simulink model "PTSD_single_channel_local_min_max_6"  (R2019b)
settings: Solver=VariableStepAuto  StartTime=0.0  StopTime=10  RelTol=1e-3
libraries: simulink x8, dspstat3 x7, dspswit3 x1
settings Model: Creator=sbuccelli  LastModifiedBy=sbuccelli

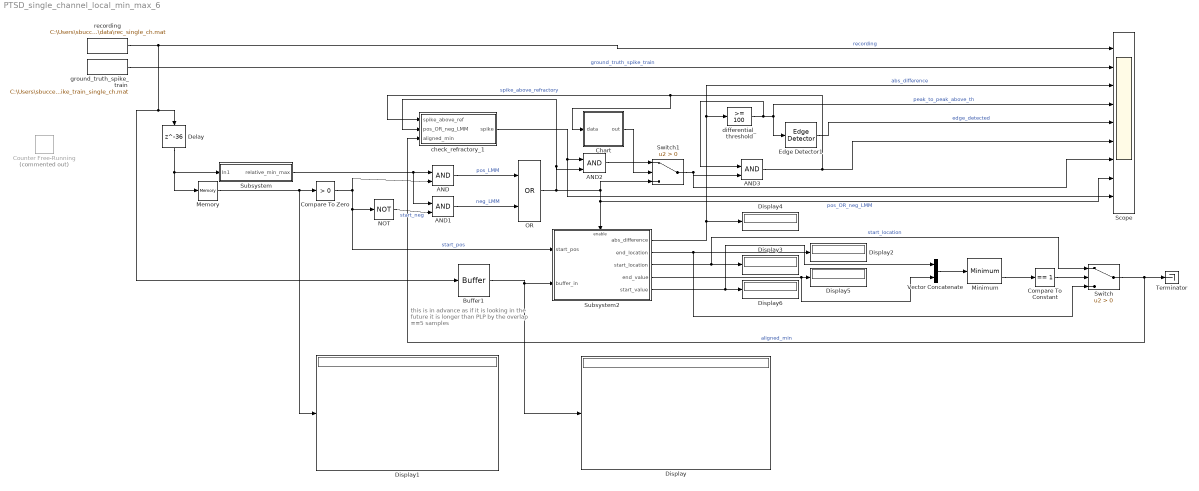
== system PTSD_single_channel_local_min_max_6 ==
  note: this is in advance as if it is looking in the future
      | it is longer than PLP by the overlap ==5 samples
  AND{,1..3} (4 alike) : Logic  IconShape=distinctive  AllPortsSameDT=off  OutDataTypeStr=boolean
  Buffer1 : Buffer  N=38  V=37  OutputFrames=off
  Chart : Stateflow chart  BlockKeywords=__PRM__SERIALIZED__DATA__:Stateflow Chart,Stateflow Diagram  TreatAsAtomicUnit=on
  Compare To Constant : simulink/Logic and Bit Operations/Compare To Constant  relop===  const=1  OutDataTypeStr=boolean
  Compare To Zero : simulink/Logic and Bit Operations/Compare To Zero  relop=>  OutDataTypeStr=boolean
  Counter Free-Running : simulink/Sources/Counter Free-Running  Commented=on  NumBits=32  tsamp=-1
  Delay : Delay  DelayLength=36
  Display{,1..6} (7 alike) : Display
  Edge Detector1 : dspswit3/Edge Detector  InputProcessing=Columns as channels (frame based)
      settings: SourceProductName=DSP System Toolbox  SourceProductBaseCode=DS
  Memory : Memory  InheritSampleTime=on
  Minimum : dspstat3/Minimum  operation=minimum  fcn=Value and Index  indexBase=One  operateOver=Each column  Dimension=1  InputProcessing=Columns as channels (frame based)  reset=None  roiEnable=off  roiType=Rectangles  roiPortion=Entire ROI  roiOutput=Individual statistics for each ROI  roiFlag=off  roundingMode=Floor  overflowMode=off
      settings: SourceProductName=DSP System Toolbox  SourceProductBaseCode=DS
  NOT : Logic  Operator=NOT  IconShape=distinctive  AllPortsSameDT=off  OutDataTypeStr=boolean
  OR : Logic  Operator=OR  IconShape=distinctive  AllPortsSameDT=off  OutDataTypeStr=boolean
  Scope : Scope  NumInputPorts=9
  Subsystem : Subsystem
  Subsystem2 : Subsystem
  Switch : Switch  Criteria=u2 > Threshold
  Switch1 : Switch  Criteria=u2 > Threshold
  Terminator : Terminator
  Vector Concatenate : Concatenate
  check_refractory_1 : Subsystem
  differential_threshold : simulink/Logic and Bit Operations/Compare To Constant  relop=>=  const=100  OutDataTypeStr=boolean
  ground_truth_spike_train : FromFile  FileName=C:\Users\sbuccelli\Documents\GitHub\closed-loop-neuroscience\data\spike_train_single_ch.mat  SampleTime=1/32e3
  recording : FromFile  FileName=C:\Users\sbuccelli\Documents\GitHub\closed-loop-neuroscience\data\rec_single_ch.mat  SampleTime=1/32e3
  wires:
  recording/1 -> Buffer1/1, Delay/1, Scope/1  "recording"
  ground_truth_spike_train/1 -> Scope/2  "ground_truth_spike_train"
  Subsystem/1(relative_min_max) -> AND/1, AND1/1
  Compare To Zero/1 -> Subsystem2/1(start_pos), NOT/1, AND/2  "start_pos"
  NOT/1 -> AND1/2  "start_neg"
  AND/1 -> OR/1  "pos_LMM"
  AND1/1 -> OR/2  "neg_LMM"
  OR/1 -> check_refractory_1/2(pos_OR_neg_LMM), AND2/2, Subsystem2/Enable, Scope/8, Switch1/3  "pos_OR_neg_LMM"
  Delay/1 -> Memory/1, Subsystem/1(In1)
  differential_threshold/1 -> AND3/1, Scope/4, Edge Detector1/1  "peak_to_peak_above_th"
  Subsystem2/1(abs_difference) -> Display4/1, Scope/3, differential_threshold/1  "abs_difference"
  Buffer1/1 -> Display/1, Subsystem2/2(buffer_in)
  Edge Detector1/1 -> Scope/5  "edge_detected"
  AND3/1 -> Scope/6, check_refractory_1/1(spike_above_ref), Chart/1(data)  "spike_above_refractory"
  Memory/1 -> Display1/1, Compare To Zero/1
  Subsystem2/2(end_location) -> Switch/3, Display2/1
  Subsystem2/4(end_value) -> Vector Concatenate/2, Display5/1
  Subsystem2/5(start_value) -> Vector Concatenate/1, Display6/1
  Subsystem2/3(start_location) -> Switch/1, Display3/1  "start_location"
  Vector Concatenate/1 -> Minimum/1
  Minimum/2 -> Compare To Constant/1
  Compare To Constant/1 -> Switch/2
  Switch/1 -> check_refractory_1/3(aligned_min), Terminator/1  "aligned_min"
  check_refractory_1/1(spike) -> Scope/9, AND2/1
  Switch1/1 -> Scope/7, AND3/2
  AND2/1 -> Switch1/1
  Chart/1(out) -> Switch1/2

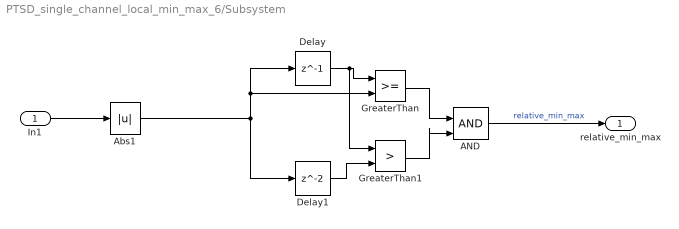
== system PTSD_single_channel_local_min_max_6/Subsystem ==
  In1 : Inport
  AND : Logic  IconShape=distinctive  AllPortsSameDT=off  OutDataTypeStr=boolean
  Abs1 : Abs
  Delay : Delay  DelayLength=1
  Delay1 : Delay
  GreaterThan : RelationalOperator  OutDataTypeStr=boolean  RndMeth=Simplest
  GreaterThan1 : RelationalOperator  Operator=>  OutDataTypeStr=boolean  RndMeth=Simplest
  relative_min_max : Outport
  wires:
  In1/1 -> Abs1/1
  Delay1/1 -> GreaterThan1/2
  GreaterThan1/1 -> AND/2
  GreaterThan/1 -> AND/1
  Delay/1 -> GreaterThan1/1, GreaterThan/1
  AND/1 -> relative_min_max/1  "relative_min_max"
  Abs1/1 -> Delay/1, GreaterThan/2, Delay1/1

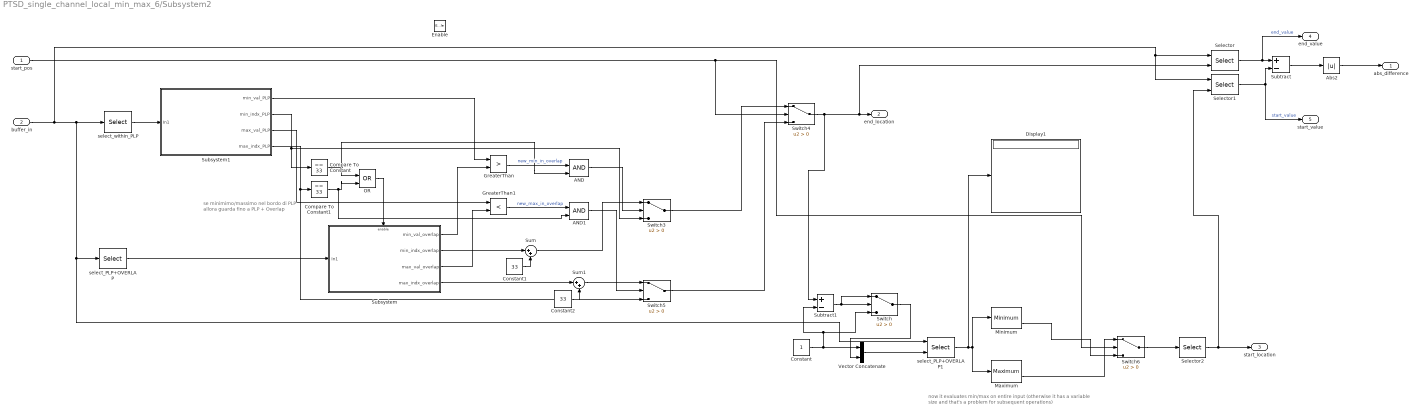
== system PTSD_single_channel_local_min_max_6/Subsystem2 ==
  note: now it evaluates min/max on entire input (otherwise it has a variable size and that's a problem for subsequent operations)
  note: se minimimo/massimo nel bordo di PLP allora guarda fino a PLP + Overlap
  start_pos : Inport
  buffer_in : Inport  Port=2
  Enable : EnablePort  PropagateVarSize=During execution
  AND : Logic  IconShape=distinctive  AllPortsSameDT=off  OutDataTypeStr=boolean
  AND1 : Logic  IconShape=distinctive  AllPortsSameDT=off  OutDataTypeStr=boolean
  Abs2 : Abs
  Compare To Constant : simulink/Logic and Bit Operations/Compare To Constant  relop===  const=33  OutDataTypeStr=boolean
  Compare To Constant1 : simulink/Logic and Bit Operations/Compare To Constant  relop===  const=33  OutDataTypeStr=boolean
  Constant : Constant
  Constant1 : Constant  Value=33
  Constant2 : Constant  Value=33
  Display1 : Display
  GreaterThan : RelationalOperator  Operator=>  OutDataTypeStr=boolean  RndMeth=Simplest
  GreaterThan1 : RelationalOperator  Operator=<  OutDataTypeStr=boolean  RndMeth=Simplest
  Maximum : dspstat3/Maximum  operation=maximum  fcn=Value and Index  indexBase=One  operateOver=Entire input  Dimension=1  InputProcessing=Columns as channels (frame based)  reset=None  roiEnable=off  roiType=Rectangles  roiPortion=Entire ROI  roiOutput=Individual statistics for each ROI  roiFlag=off  roundingMode=Floor  overflowMode=off  accumDataTypeStr=Inherit: Same as product output  accumLastDataTypeStr=Inherit: Same as product output
  Minimum : dspstat3/Minimum  operation=minimum  fcn=Value and Index  indexBase=One  operateOver=Entire input  Dimension=1  InputProcessing=Columns as channels (frame based)  reset=None  roiEnable=off  roiType=Rectangles  roiPortion=Entire ROI  roiOutput=Individual statistics for each ROI  roiFlag=off  roundingMode=Floor  overflowMode=off
      settings: SourceProductName=DSP System Toolbox  SourceProductBaseCode=DS
  OR : Logic  Operator=OR  IconShape=distinctive  AllPortsSameDT=off  OutDataTypeStr=boolean
  Selector : Selector  IndexOptions=Index vector (port)  Indices=[1 3]  OutputSizes=1
  Selector1 : Selector  IndexOptions=Index vector (port)  Indices=[1 3]  OutputSizes=1
  Selector2 : Selector  NumberOfDimensions=2  IndexOptions=Select all,Index vector (dialog)  Indices=[1 3],1  OutputSizes=1,1
  Subsystem : Subsystem
  Subsystem1 : Subsystem
  Subtract : Sum  Inputs=+-
  Subtract1 : Sum  Inputs=+-
  Sum : Sum  Inputs=|++
  Sum1 : Sum  Inputs=|++
  Switch{,3..6} (5 alike) : Switch  Criteria=u2 > Threshold
  Vector Concatenate : Concatenate
  select_PLP+OVERLAP : Selector  NumberOfDimensions=2  InputPortWidth=3  IndexOptions=Index vector (dialog),Index vector (dialog)  Indices=[34:38],1  OutputSizes=1,1
  select_PLP+OVERLAP1 : Selector  NumberOfDimensions=2  InputPortWidth=3  IndexOptions=Starting and ending indices (port),Index vector (dialog)  Indices=[25:29],1  OutputSizes=1,1
  select_within_PLP : Selector  NumberOfDimensions=2  InputPortWidth=3  IndexOptions=Index vector (dialog),Index vector (dialog)  Indices=[1:33],1  OutputSizes=1,1
  abs_difference : Outport
  end_location : Outport  Port=2
  start_location : Outport  Port=3
  end_value : Outport  Port=4
  start_value : Outport  Port=5
  wires:
  Abs2/1 -> abs_difference/1
  buffer_in/1 -> Selector1/1, Selector/1, select_within_PLP/1, select_PLP+OVERLAP1/1, select_PLP+OVERLAP/1
  Subtract/1 -> Abs2/1
  Compare To Constant/1 -> OR/1, AND/2
  Compare To Constant1/1 -> AND1/2, OR/2
  OR/1 -> Subsystem/Enable
  select_PLP+OVERLAP/1 -> Subsystem/1(In1)
  select_within_PLP/1 -> Subsystem1/1(In1)
  Subsystem1/2(min_indx_PLP) -> Switch3/3, Compare To Constant/1
  Subsystem1/4(max_indx_PLP) -> Switch5/3, Compare To Constant1/1
  Subsystem1/1(min_val_PLP) -> GreaterThan/1
  Subsystem/1(min_val_overlap) -> GreaterThan/2
  Subsystem1/3(max_val_PLP) -> GreaterThan1/1
  Subsystem/3(max_val_overlap) -> GreaterThan1/2
  GreaterThan/1 -> AND/1  "new_min_in_overlap"
  GreaterThan1/1 -> AND1/1  "new_max_in_overlap"
  AND/1 -> Switch3/2
  AND1/1 -> Switch5/2
  Switch3/1 -> Switch4/1
  Switch5/1 -> Switch4/3
  Vector Concatenate/1 -> select_PLP+OVERLAP1/2
  start_pos/1 -> Switch4/2, Switch6/2
  select_PLP+OVERLAP1/1 -> Display1/1, Maximum/1, Minimum/1
  Minimum/2 -> Switch6/3
  Maximum/2 -> Switch6/1
  Selector/1 -> end_value/1, Subtract/1  "end_value"
  Selector1/1 -> start_value/1, Subtract/2  "start_value"
  Switch4/1 -> Selector/2, end_location/1, Subtract1/1
  Switch6/1 -> Selector2/1
  Selector2/1 -> start_location/1, Selector1/2
  Subtract1/1 -> Switch/1, Switch/2
  Constant/1 -> Vector Concatenate/1, Switch/3, Subtract1/2
  Switch/1 -> Vector Concatenate/2
  Subsystem/2(min_indx_overlap) -> Sum/1
  Sum/1 -> Switch3/1
  Constant1/1 -> Sum/2
  Subsystem/4(max_indx_overlap) -> Sum1/1
  Constant2/1 -> Sum1/2
  Sum1/1 -> Switch5/1

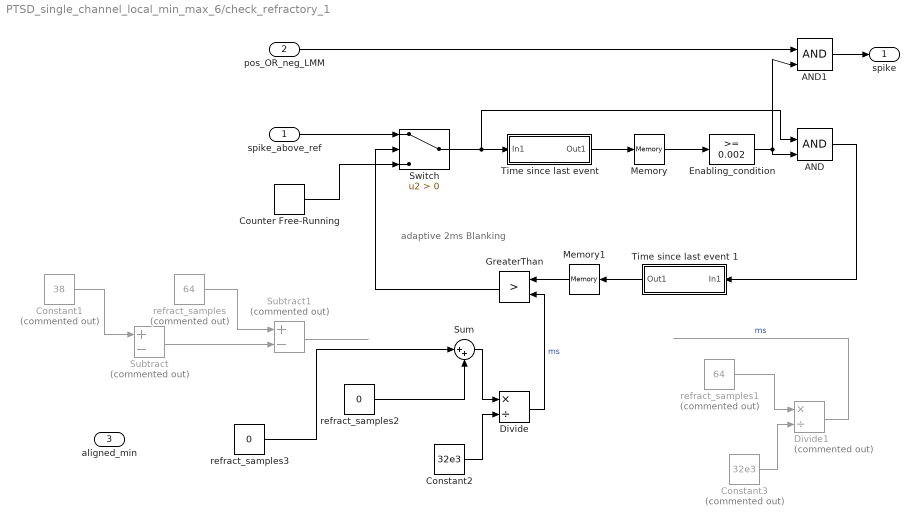
== system PTSD_single_channel_local_min_max_6/check_refractory_1 ==
  note: adaptive 2ms Blanking
  spike_above_ref : Inport
  pos_OR_neg_LMM : Inport  Port=2
  aligned_min : Inport  Port=3
  AND : Logic  IconShape=distinctive  AllPortsSameDT=off  OutDataTypeStr=boolean
  AND1 : Logic  IconShape=distinctive  AllPortsSameDT=off  OutDataTypeStr=boolean
  Constant1 : Constant  Commented=on  Value=38
  Constant2 : Constant  Value=32e3
  Constant3 : Constant  Commented=on  Value=32e3
  Counter Free-Running : simulink/Sources/Counter Free-Running  NumBits=1  tsamp=-1
  Divide : Product  Inputs=*/
  Divide1 : Product  Commented=on  Inputs=*/
  Enabling_condition : simulink/Logic and Bit Operations/Compare To Constant  relop=>=  const=0.002  OutDataTypeStr=boolean
  GreaterThan : RelationalOperator  Operator=>  OutDataTypeStr=boolean  RndMeth=Simplest
  Memory : Memory  InheritSampleTime=on
  Memory1 : Memory  InheritSampleTime=on
  Subtract : Sum  Commented=on  Inputs=+-
  Subtract1 : Sum  Commented=on  Inputs=+-
  Sum : Sum  Inputs=|++
  Switch : Switch  Criteria=u2 > Threshold
  "Time since last event " : Subsystem
  Time since last event 1 : Subsystem
  refract_samples : Constant  Commented=on  Value=64
  refract_samples1 : Constant  Commented=on  Value=64
  refract_samples2 : Constant  Value=0
  refract_samples3 : Constant  Value=0
  spike : Outport
  wires:
  Memory/1 -> Enabling_condition/1
  "Time since last event "/1(Out1) -> Memory/1
  Time since last event 1/1(Out1) -> Memory1/1
  Counter Free-Running/1 -> Switch/3
  GreaterThan/1 -> Switch/2
  spike_above_ref/1 -> Switch/1
  Switch/1 -> AND/1, "Time since last event "/1(In1)
  Constant1/1 -> Subtract/1
  Subtract/1 -> Subtract1/2
  refract_samples/1 -> Subtract1/1
  Subtract1/1 -> ?
  Constant2/1 -> Divide/2
  Divide/1 -> GreaterThan/2  "ms"
  AND/1 -> Time since last event 1/1(In1)
  Enabling_condition/1 -> AND1/2, AND/2
  pos_OR_neg_LMM/1 -> AND1/1
  AND1/1 -> spike/1
  refract_samples1/1 -> Divide1/1
  Constant3/1 -> Divide1/2
  Divide1/1 -> ?  "ms"
  Sum/1 -> Divide/1
  refract_samples2/1 -> Sum/2
  refract_samples3/1 -> Sum/1
  Memory1/1 -> GreaterThan/1

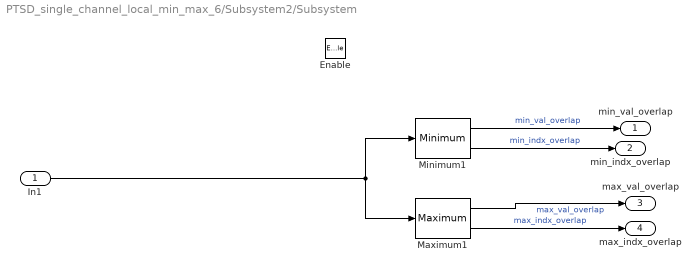
== system PTSD_single_channel_local_min_max_6/Subsystem2/Subsystem ==
  In1 : Inport
  Enable : EnablePort
  Maximum1 : dspstat3/Maximum  operation=maximum  fcn=Value and Index  indexBase=One  operateOver=Each column  Dimension=1  InputProcessing=Columns as channels (frame based)  reset=None  roiEnable=off  roiType=Rectangles  roiPortion=Entire ROI  roiOutput=Individual statistics for each ROI  roiFlag=off  roundingMode=Floor  overflowMode=off  accumDataTypeStr=Inherit: Same as product output  accumLastDataTypeStr=Inherit: Same as product output
  Minimum1 : dspstat3/Minimum  operation=minimum  fcn=Value and Index  indexBase=One  operateOver=Each column  Dimension=1  InputProcessing=Columns as channels (frame based)  reset=None  roiEnable=off  roiType=Rectangles  roiPortion=Entire ROI  roiOutput=Individual statistics for each ROI  roiFlag=off  roundingMode=Floor  overflowMode=off
      settings: SourceProductName=DSP System Toolbox  SourceProductBaseCode=DS
  min_val_overlap : Outport
  min_indx_overlap : Outport  Port=2
  max_val_overlap : Outport  Port=3
  max_indx_overlap : Outport  Port=4
  wires:
  Minimum1/2 -> min_indx_overlap/1  "min_indx_overlap"
  In1/1 -> Minimum1/1, Maximum1/1
  Maximum1/2 -> max_indx_overlap/1  "max_indx_overlap"
  Minimum1/1 -> min_val_overlap/1  "min_val_overlap"
  Maximum1/1 -> max_val_overlap/1  "max_val_overlap"

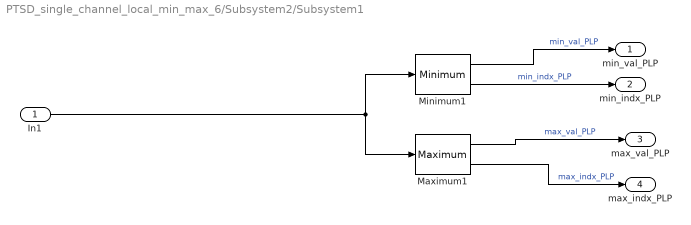
== system PTSD_single_channel_local_min_max_6/Subsystem2/Subsystem1 ==
  In1 : Inport
  Maximum1 : dspstat3/Maximum  operation=maximum  fcn=Value and Index  indexBase=One  operateOver=Each column  Dimension=1  InputProcessing=Columns as channels (frame based)  reset=None  roiEnable=off  roiType=Rectangles  roiPortion=Entire ROI  roiOutput=Individual statistics for each ROI  roiFlag=off  roundingMode=Floor  overflowMode=off  accumDataTypeStr=Inherit: Same as product output  accumLastDataTypeStr=Inherit: Same as product output
  Minimum1 : dspstat3/Minimum  operation=minimum  fcn=Value and Index  indexBase=One  operateOver=Each column  Dimension=1  InputProcessing=Columns as channels (frame based)  reset=None  roiEnable=off  roiType=Rectangles  roiPortion=Entire ROI  roiOutput=Individual statistics for each ROI  roiFlag=off  roundingMode=Floor  overflowMode=off
      settings: SourceProductName=DSP System Toolbox  SourceProductBaseCode=DS
  min_val_PLP : Outport
  min_indx_PLP : Outport  Port=2
  max_val_PLP : Outport  Port=3
  max_indx_PLP : Outport  Port=4
  wires:
  Minimum1/2 -> min_indx_PLP/1  "min_indx_PLP"
  In1/1 -> Minimum1/1, Maximum1/1
  Maximum1/2 -> max_indx_PLP/1  "max_indx_PLP"
  Minimum1/1 -> min_val_PLP/1  "min_val_PLP"
  Maximum1/1 -> max_val_PLP/1  "max_val_PLP"

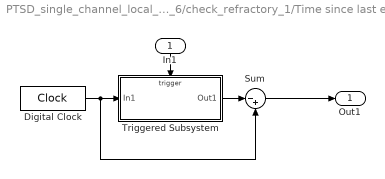
== system PTSD_single_channel_local_min_max_6/check_refractory_1/Time since last event  ==
  In1 : Inport
  Digital Clock : DigitalClock  SampleTime=1/32e3
  Sum : Sum  Inputs=|-+
  Triggered Subsystem : Subsystem  TreatAsAtomicUnit=on
  Out1 : Outport
  wires:
  Digital Clock/1 -> Sum/2, Triggered Subsystem/1(In1)
  Triggered Subsystem/1(Out1) -> Sum/1
  In1/1 -> Triggered Subsystem/Trigger
  Sum/1 -> Out1/1

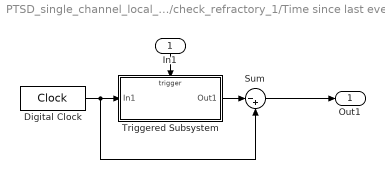
== system PTSD_single_channel_local_min_max_6/check_refractory_1/Time since last event 1 ==
  In1 : Inport
  Digital Clock : DigitalClock  SampleTime=1/32e3
  Sum : Sum  Inputs=|-+
  Triggered Subsystem : Subsystem  TreatAsAtomicUnit=on
  Out1 : Outport
  wires:
  Digital Clock/1 -> Sum/2, Triggered Subsystem/1(In1)
  Triggered Subsystem/1(Out1) -> Sum/1
  In1/1 -> Triggered Subsystem/Trigger
  Sum/1 -> Out1/1

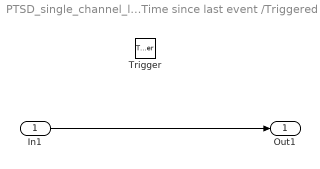
== system PTSD_single_channel_local_min_max_6/check_refractory_1/Time since last event /Triggered Subsystem ==
  In1 : Inport
  Trigger : TriggerPort  VariantControl=Variant
  Out1 : Outport
  wires:
  In1/1 -> Out1/1

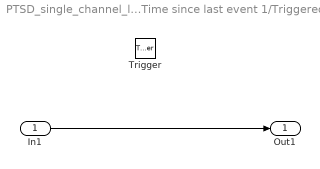
== system PTSD_single_channel_local_min_max_6/check_refractory_1/Time since last event 1/Triggered Subsystem ==
  In1 : Inport
  Trigger : TriggerPort  VariantControl=Variant
  Out1 : Outport
  wires:
  In1/1 -> Out1/1

== stateflow chart PTSD_single_channel_local_min_max_6/Chart ==
  settings: stateMachineType=MOORE_MACHINE
  state zero
    out=0
  state zero1
    out=1
  (default) -> zero
  zero -> zero1 : [data==1]
  data: data input; out output
